simulink model "deneme"  (R2020b)
settings: Solver=VariableStepAuto  StartTime=0.0  StopTime=0.01  RelTol=1e-3
undefined symbols (not defined in the file): magnitude
libraries: dspstat3 x9, commrflib2 x2, commfilt2 x2
settings Model: Creator=erd  LastModifiedBy=Marco Ceran

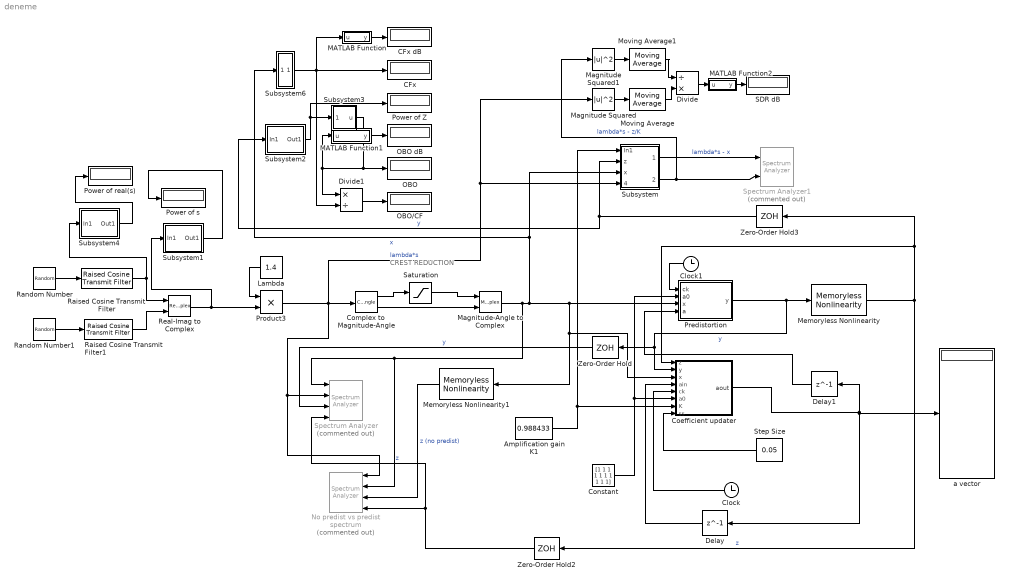
== system deneme ==
  note: CREST REDUCTION
  " CFx" : Display
  " CFx dB" : Display
  " OBO" : Display
  " OBO dB" : Display
  " OBO/CF" : Display
  " Power of Z" : Display
  " Power of real(s)" : Display
  " Power of s" : Display
  Amplification gain K1 : Constant  Value=0.988433
  Clock : Clock
  Clock1 : Clock
  Coefficient updater : MATLAB Function  TreatAsAtomicUnit=on
  Complex to Magnitude-Angle : ComplexToMagnitudeAngle
  Constant : Constant  Value=[1 1 1 1 1 1 1 1 1 1]
  Delay : Delay  DelayLength=1  InitialCondition=0
  Delay1 : Delay  DelayLength=1  InitialCondition=0
  Divide : Product  Inputs=/*
  Divide1 : Product  Inputs=*/
  Lambda : Constant  Value=1.4
  MATLAB Function : MATLAB Function  TreatAsAtomicUnit=on
  MATLAB Function1 : MATLAB Function  TreatAsAtomicUnit=on
  MATLAB Function2 : MATLAB Function  TreatAsAtomicUnit=on
  Magnitude Squared : Math  Operator=magnitude^2  SaturateOnIntegerOverflow=on
  Magnitude Squared1 : Math  Operator=magnitude^2  SaturateOnIntegerOverflow=on
  Magnitude-Angle to Complex : MagnitudeAngleToComplex
  Memoryless Nonlinearity : commrflib2/Memoryless Nonlinearity  model_select=Rapp model  linGaindB=0  GindB=0  iip3=30  am2pm=10  LPwrLimAMPM=10  UPwrLimAMPM=inf  amam=[2.1587 1.1517]  ampm=[4.0033 9.1040]  x=[8.1081 1.5413 6.5202 -0.0718]  y=[4.6645 2.0965 10.88 -0.003]  p=2.5  GoutdB=0  vsat=1
      settings: SourceProductBaseCode=CM
  Memoryless Nonlinearity1 : commrflib2/Memoryless Nonlinearity  model_select=Rapp model  linGaindB=0  GindB=0  iip3=30  am2pm=10  LPwrLimAMPM=10  UPwrLimAMPM=inf  amam=[2.1587 1.1517]  ampm=[4.0033 9.1040]  x=[8.1081 1.5413 6.5202 -0.0718]  y=[4.6645 2.0965 10.88 -0.003]  p=2.5  GoutdB=0  vsat=1
      settings: SourceProductBaseCode=CM
  Moving Average : dspstat3/Moving Average  Method=Sliding window  ForgettingFactorPort=off  SpecifyWindowLength=on  WindowLength=1000000  ForgettingFactor=0.9  SimulateUsing=Code generation
  Moving Average1 : dspstat3/Moving Average  Method=Sliding window  ForgettingFactorPort=off  SpecifyWindowLength=on  WindowLength=1000000  ForgettingFactor=0.9  SimulateUsing=Code generation
  No predist vs predist spectrum : SpectrumAnalyzer  Commented=on  NumInputPorts=4
  Predistortion : MATLAB Function  TreatAsAtomicUnit=on
  Product3 : Product
  Raised Cosine Transmit Filter : commfilt2/Raised Cosine Transmit Filter  filtType=Square root  R=0.2  filtSpan=80  N=8  filterGain=1  InputProcessing=Columns as channels (frame based)  RateOptions=Enforce single-rate processing  framing=Mute  checkCoeff=off  variableName=rcTxFilt  checkGain=Normalized  sampMode=Mute  saveAsFlag=0  currentFiltSpan=80  D=(80)/2  launchFVT=on  roundingMode=Floor  overflowMode=off  coeffDataTypeStr=Inherit: Same word length as input  coeffMin=[]  coeffMax=[]  coeffLastDataTypeStr=Inherit: Same word length as input  outputDataTypeStr=Inherit: Same as accumulator  outputMin=[]  outputMax=[]  outputLastDataTypeStr=Inherit: Same as accumulator
  Raised Cosine Transmit Filter1 : commfilt2/Raised Cosine Transmit Filter  filtType=Square root  R=0.2  filtSpan=80  N=8  filterGain=1  InputProcessing=Columns as channels (frame based)  RateOptions=Enforce single-rate processing  framing=Mute  checkCoeff=off  variableName=rcTxFilt1  checkGain=Normalized  sampMode=Mute  saveAsFlag=0  currentFiltSpan=80  D=(80)/2  launchFVT=on  roundingMode=Floor  overflowMode=off  coeffDataTypeStr=Inherit: Same word length as input  coeffMin=[]  coeffMax=[]  coeffLastDataTypeStr=Inherit: Same word length as input  outputDataTypeStr=Inherit: Same as accumulator  outputMin=[]  outputMax=[]  outputLastDataTypeStr=Inherit: Same as accumulator
  Random Number : RandomNumber  Seed=3  SampleTime=0.0000002
  Random Number1 : RandomNumber  Seed=4  SampleTime=0.0000002
  Real-Imag to Complex : RealImagToComplex
  SDR dB : Display
  Saturation : Saturate  UpperLimit=1  LowerLimit=0  LinearizeAsGain=off
  Spectrum Analyzer : SpectrumAnalyzer  Commented=on  NumInputPorts=4
  Spectrum Analyzer1 : SpectrumAnalyzer  Commented=on  NumInputPorts=2
  Step Size : Constant  Value=0.05
  Subsystem : Subsystem
  Subsystem1 : Subsystem
  Subsystem2 : Subsystem
  Subsystem3 : Subsystem
  Subsystem4 : Subsystem
  Subsystem6 : Subsystem
  Zero-Order Hold : ZeroOrderHold  SampleTime=-1
  Zero-Order Hold2 : ZeroOrderHold  SampleTime=-1
  Zero-Order Hold3 : ZeroOrderHold  SampleTime=-1
  a vector : Display
  wires:
  Complex to Magnitude-Angle/1 -> Saturation/1
  Complex to Magnitude-Angle/2 -> Magnitude-Angle to Complex/2
  Saturation/1 -> Magnitude-Angle to Complex/1
  Random Number1/1 -> Raised Cosine Transmit Filter1/1
  Random Number/1 -> Raised Cosine Transmit Filter/1
  Memoryless Nonlinearity/1 -> Coefficient updater/1(z), Zero-Order Hold3/1, Zero-Order Hold2/1  "z"
  Step Size/1 -> Coefficient updater/8(ss)
  Clock/1 -> Coefficient updater/5(ck)
  Constant/1 -> Predistortion/2(a0), Coefficient updater/6(a0)
  Clock1/1 -> Predistortion/1(ck)
  Product3/1 -> Subsystem/4(lambda*s), Magnitude Squared/1, No predist vs predist spectrum/1, Spectrum Analyzer/2, Complex to Magnitude-Angle/1  "lambda*s"
  Lambda/1 -> Product3/1
  Magnitude-Angle to Complex/1 -> No predist vs predist spectrum/2, Spectrum Analyzer/1, Memoryless Nonlinearity1/1, Coefficient updater/3(x), Predistortion/3(x), Subsystem/3(x), Subsystem6/1(In1)  "x"
  MATLAB Function1/1(y) -> " OBO dB"/1
  MATLAB Function/1(y) -> " CFx dB"/1
  Divide1/1 -> " OBO/CF"/1
  Subsystem6/1(u) -> Divide1/2, MATLAB Function/1(u), " CFx"/1
  Subsystem3/1(u) -> MATLAB Function1/1(u), Divide1/1, " OBO"/1
  Subsystem2/1(Out1) -> " Power of Z"/1, Subsystem3/1(In1)
  Memoryless Nonlinearity1/1 -> No predist vs predist spectrum/3  "z (no predist)"
  Predistortion/1(y) -> Memoryless Nonlinearity/1, Zero-Order Hold/1, Coefficient updater/2(y)  "y"
  Amplification gain K1/1 -> Subsystem/1(In1), Coefficient updater/7(K)
  Subsystem/2(Out2) -> Spectrum Analyzer1/2, Magnitude Squared1/1  "lambda*s - z/K"
  Coefficient updater/1(aout) -> a vector/1, Delay/1, Delay1/1
  Delay/1 -> Coefficient updater/4(ain)
  Zero-Order Hold/1 -> Spectrum Analyzer/3  "y"
  Zero-Order Hold2/1 -> No predist vs predist spectrum/4, Spectrum Analyzer/4  "z"
  Zero-Order Hold3/1 -> Subsystem/2(z), Subsystem2/1(In1)  "y"
  Subsystem1/1(Out1) -> " Power of s"/1
  Real-Imag to Complex/1 -> Subsystem1/1(In1), Product3/2
  Subsystem4/1(Out1) -> " Power of real(s)"/1
  Raised Cosine Transmit Filter/1 -> Subsystem4/1(In1), Real-Imag to Complex/1
  Divide/1 -> MATLAB Function2/1(u)
  MATLAB Function2/1(y) -> SDR dB/1
  Magnitude Squared/1 -> Moving Average/1
  Magnitude Squared1/1 -> Moving Average1/1
  Moving Average1/1 -> Divide/1
  Moving Average/1 -> Divide/2
  Subsystem/1(Out1) -> Spectrum Analyzer1/1  "lambda*s - x"
  Delay1/1 -> Predistortion/4(a)
  Raised Cosine Transmit Filter1/1 -> Real-Imag to Complex/2

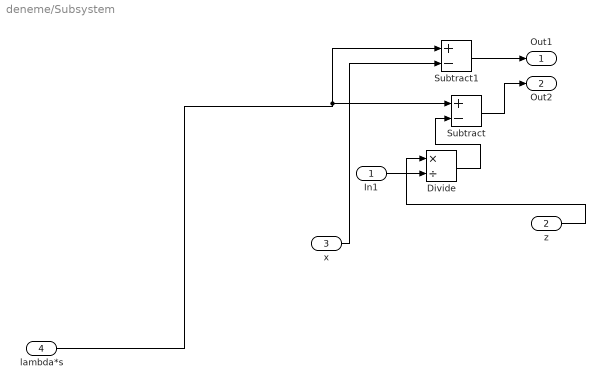
== system deneme/Subsystem ==
  In1 : Inport
  z : Inport  Port=2
  x : Inport  Port=3
  lambda*s : Inport  Port=4
  Divide : Product  Inputs=*/
  Subtract : Sum  Inputs=+-
  Subtract1 : Sum  Inputs=+-
  Out1 : Outport
  Out2 : Outport  Port=2
  wires:
  Subtract/1 -> Out2/1
  Divide/1 -> Subtract/2
  z/1 -> Divide/1
  lambda*s/1 -> Subtract1/1, Subtract/1
  x/1 -> Subtract1/2
  Subtract1/1 -> Out1/1
  In1/1 -> Divide/2

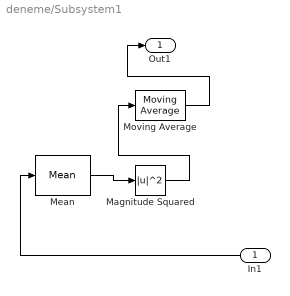
== system deneme/Subsystem1 ==
  In1 : Inport
  Magnitude Squared : Math  Operator=magnitude^2  SaturateOnIntegerOverflow=on
  Mean : dspstat3/Mean  run=off  InputProcessing=Columns as channels (frame based)  reset_popup=None  directionMode=Each column  dimension=1  roiEnable=off  roiType=Rectangles  roiPortion=Entire ROI  roiOutput=Individual statistics for each ROI  roiFlag=off  roundingMode=Floor  overflowMode=off  outputDataTypeStr=Inherit: Same as accumulator  outputMin=[]  outputMax=[]  outputLastDataTypeStr=Inherit: Same as accumulator
  Moving Average : dspstat3/Moving Average  Method=Sliding window  ForgettingFactorPort=off  SpecifyWindowLength=on  WindowLength=1500  ForgettingFactor=0.9  SimulateUsing=Code generation
  Out1 : Outport
  wires:
  Magnitude Squared/1 -> Moving Average/1
  Moving Average/1 -> Out1/1
  Mean/1 -> Magnitude Squared/1
  In1/1 -> Mean/1

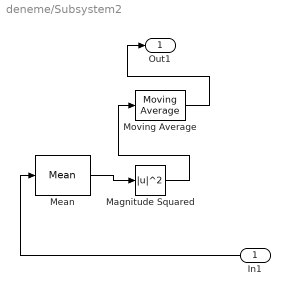
== system deneme/Subsystem2 ==
  In1 : Inport
  Magnitude Squared : Math  Operator=magnitude^2  SaturateOnIntegerOverflow=on
  Mean : dspstat3/Mean  run=off  InputProcessing=Columns as channels (frame based)  reset_popup=None  directionMode=Each column  dimension=1  roiEnable=off  roiType=Rectangles  roiPortion=Entire ROI  roiOutput=Individual statistics for each ROI  roiFlag=off  roundingMode=Floor  overflowMode=off  outputDataTypeStr=Inherit: Same as accumulator  outputMin=[]  outputMax=[]  outputLastDataTypeStr=Inherit: Same as accumulator
  Moving Average : dspstat3/Moving Average  Method=Sliding window  ForgettingFactorPort=off  SpecifyWindowLength=on  WindowLength=1500  ForgettingFactor=0.9  SimulateUsing=Code generation
  Out1 : Outport
  wires:
  Magnitude Squared/1 -> Moving Average/1
  Moving Average/1 -> Out1/1
  Mean/1 -> Magnitude Squared/1
  In1/1 -> Mean/1

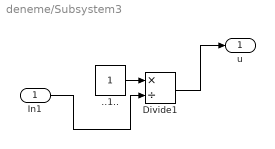
== system deneme/Subsystem3 ==
  In1 : Inport
  ..1.. : Constant
  Divide1 : Product  Inputs=*/
  u : Outport
  wires:
  ..1../1 -> Divide1/1
  In1/1 -> Divide1/2
  Divide1/1 -> u/1

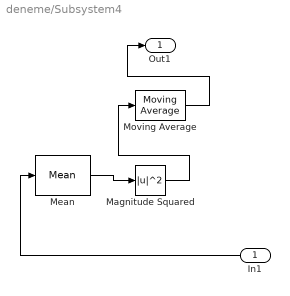
== system deneme/Subsystem4 ==
  In1 : Inport
  Magnitude Squared : Math  Operator=magnitude^2  SaturateOnIntegerOverflow=on
  Mean : dspstat3/Mean  run=off  InputProcessing=Columns as channels (frame based)  reset_popup=None  directionMode=Each column  dimension=1  roiEnable=off  roiType=Rectangles  roiPortion=Entire ROI  roiOutput=Individual statistics for each ROI  roiFlag=off  roundingMode=Floor  overflowMode=off  outputDataTypeStr=Inherit: Same as accumulator  outputMin=[]  outputMax=[]  outputLastDataTypeStr=Inherit: Same as accumulator
  Moving Average : dspstat3/Moving Average  Method=Sliding window  ForgettingFactorPort=off  SpecifyWindowLength=on  WindowLength=1500  ForgettingFactor=0.9  SimulateUsing=Code generation
  Out1 : Outport
  wires:
  Magnitude Squared/1 -> Moving Average/1
  Moving Average/1 -> Out1/1
  Mean/1 -> Magnitude Squared/1
  In1/1 -> Mean/1

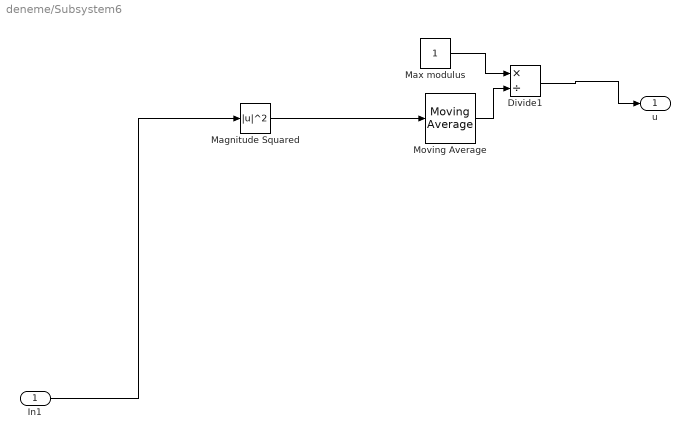
== system deneme/Subsystem6 ==
  In1 : Inport
  Divide1 : Product  Inputs=*/
  Magnitude Squared : Math  Operator=magnitude^2  SaturateOnIntegerOverflow=on
  Max modulus : Constant
  Moving Average : dspstat3/Moving Average  Method=Sliding window  ForgettingFactorPort=off  SpecifyWindowLength=on  WindowLength=50000  ForgettingFactor=0.9  SimulateUsing=Code generation
  u : Outport
  wires:
  Max modulus/1 -> Divide1/1
  Moving Average/1 -> Divide1/2
  In1/1 -> Magnitude Squared/1
  Divide1/1 -> u/1
  Magnitude Squared/1 -> Moving Average/1

== matlab function deneme/Predistortion ==
  data: ck input; a0 input; x input; y output; a input
function y = predistort(ck, a0, x, a)
if ck == 0
   aa = a0;
else aa = a;
end
N = length(aa);
outpt = x-x;
for j = 1:length(x)
    for k = 1:(N-1)
        if (abs(x(j))>=1)
            outpt(j) = x(j)*a(end);
        end
        if (k-1)/(N-1) <= abs(x(j)) && k/(N-1) > abs(x(j))
            outpt(j) = x(j)*(aa(k+1)+(a(k+1)-a(k))*(abs(x(j))*(N-1)-k));
            %outpt(j) = (aa(k) + (aa(k+1)-aa(k))*(abs(x(j))*(N-1)-k+1));
        end
    end
end
y = outpt;

== matlab function deneme/MATLAB Function2 ==
  data: u input; y output
function y = lintodb(u)
y = mean(10.*log10(u));

== matlab function deneme/Coefficient updater ==
  data: z input; y input; x input; ain input; ck input; a0 input; aout output; K input; ss input
function aout = adapt(z, y, x, ain, ck, a0, K, ss)
if ck < 5e-6
    aout = a0;
else
aux = ain;  %auxiliary vector
aaaa = 0;
N = length(ain);
for j = 1:length(x) % x, y and z all have the same length (8)
    for k = 1:N
        if abs(x(j)) < ((2*k-1)/(2*N-2))
            aux(k) = real(ain(k) - ss*k*(z(j)-K*x(j))*conj(z(j))*conj(x(j))/conj(y(j)));
        end
    end
end
aout = aux;
end

== matlab function deneme/MATLAB Function ==
  data: u input; y output
function y = lintodb(u)
y = mean(10.*log10(u));

== matlab function deneme/MATLAB Function1 ==
  data: u input; y output
function y = lintodb(u)
y = 10*log10(u);
